simulink model "simulink_test1"  (R2014a)
settings: Solver=ode45  StartTime=0.0  StopTime=10.0  RelTol=1e-3
values from neighbouring files (symbols this model uses):
  Gb = 200    [pole_placement.m]    (also in pole_placement2.m; time_domain.m)
  Ib = 0    [pole_placement.m]    (also in pole_placement2.m; time_domain.m)
  n = 0.142    [pole_placement.m]    (also in pole_placement2.m; time_domain.m)
  p1 = 0.035    [pole_placement.m]    (also in pole_placement2.m; time_domain.m)
  p2 = 0.05    [pole_placement.m]    (also in pole_placement2.m; time_domain.m)
  p3 = 0.000023    (= 2.3e-05)    [pole_placement.m]    (also in pole_placement2.m = 2.8e-05; time_domain.m)
  VG = 117    [pole_placement.m]    (also in pole_placement2.m; time_domain.m)
  VI = 1/0.098    (= 10.2040816327)    [pole_placement.m]    (also in pole_placement2.m; time_domain.m)
undefined symbols (not defined in the file or in its folder): Ge, k1, k2, k3, kr, l1, l2, l3, r, Vg, Xe
settings Model: Creator=joach  LastModifiedBy=joach
settings OptimizationCC: SimCompilerOptimization=off
settings DebuggingCC: MergeDetectMultiDrivingBlocksExec=error  FrameProcessingCompatibilityMsg=error
settings RTWCC: RTWCompilerOptimization=off
settings ConfigComp: CovMetricSettings=dw  CovHtmlReporting=on  CovSaveCumulativeToWorkspaceVar=on  CovSaveSingleToWorkspaceVar=on  CovModelRefEnable=Off  CovExternalEMLEnable=off  CovSFcnEnable=off

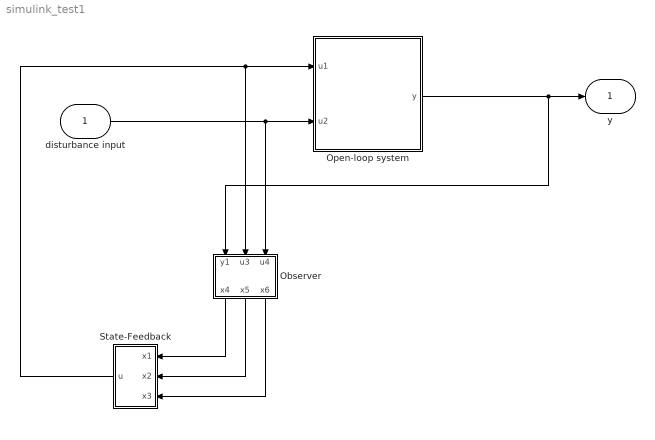
== system simulink_test1 ==
  disturbance input : Inport
  Observer : Subsystem
  Open-loop system : Subsystem
  State-Feedback : Subsystem
  y : Outport
  wires:
  disturbance input/1 -> Open-loop system/2(u2), Observer/3(u4)
  Observer/2(x5) -> State-Feedback/2(x2)
  Observer/3(x6) -> State-Feedback/3(x3)
  Open-loop system/1(y) -> Observer/1(y1), y/1
  State-Feedback/1(u) -> Open-loop system/1(u1), Observer/2(u3)
  Observer/1(x4) -> State-Feedback/1(x1)

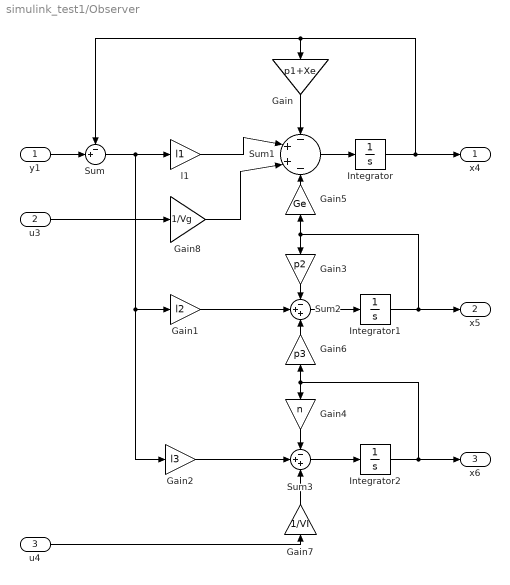
== system simulink_test1/Observer ==
  y1 : Inport
  u3 : Inport  Port=2
  u4 : Inport  Port=3
  Gain : Gain  Gain=p1+Xe
  Gain1 : Gain  Gain=l2
  Gain2 : Gain  Gain=l3
  Gain3 : Gain  Gain=p2
  Gain4 : Gain  Gain=n
  Gain5 : Gain  Gain=Ge
  Gain6 : Gain  Gain=p3
  Gain7 : Gain  Gain=1/VI
  Gain8 : Gain  Gain=1/Vg
  Integrator : Integrator
  Integrator1 : Integrator
  Integrator2 : Integrator
  Sum : Sum  Inputs=-+|
  Sum1 : Sum  Inputs=-++-
  Sum2 : Sum  Inputs=-++
  Sum3 : Sum  Inputs=-++
  l1 : Gain  Gain=l1
  x4 : Outport
  x5 : Outport  Port=2
  x6 : Outport  Port=3
  wires:
  Sum/1 -> Gain2/1, Gain1/1, l1/1
  Sum1/1 -> Integrator/1
  l1/1 -> Sum1/2
  Integrator/1 -> x4/1, Sum/1, Gain/1
  Gain2/1 -> Sum3/2
  Gain1/1 -> Sum2/2
  Integrator1/1 -> x5/1, Gain5/1, Gain3/1
  y1/1 -> Sum/2
  Gain/1 -> Sum1/1
  Sum2/1 -> Integrator1/1
  Integrator2/1 -> x6/1, Gain6/1, Gain4/1
  Gain3/1 -> Sum2/1
  Sum3/1 -> Integrator2/1
  Gain7/1 -> Sum3/3
  Gain4/1 -> Sum3/1
  Gain6/1 -> Sum2/3
  u3/1 -> Gain8/1
  Gain5/1 -> Sum1/4
  Gain8/1 -> Sum1/3
  u4/1 -> Gain7/1

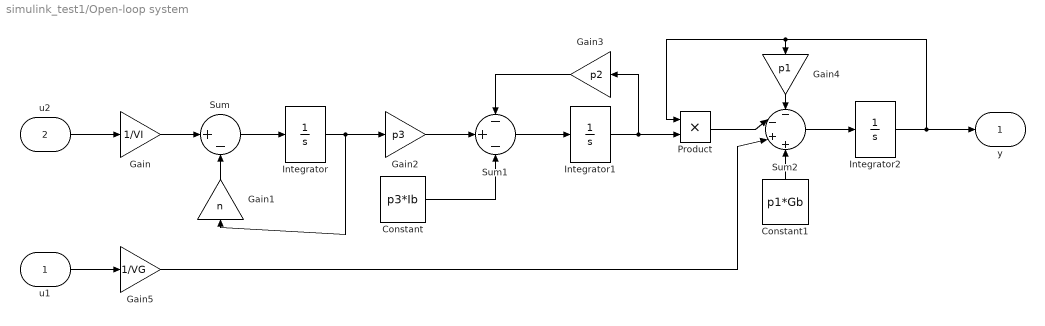
== system simulink_test1/Open-loop system ==
  u1 : Inport
  u2 : Inport  Port=2
  " Gain" : Gain  Gain=1/VI
  " Gain2" : Gain  Gain=p3
  " Gain3" : Gain  Gain=p2
  " Gain4" : Gain  Gain=p1
  " Gain5" : Gain  Gain=1/VG
  Constant : Constant  Value=p3*Ib
  Constant1 : Constant  Value=p1*Gb
  Gain1 : Gain  Gain=n
  Integrator : Integrator
  Integrator1 : Integrator
  Integrator2 : Integrator
  Product : Product
  Sum : Sum  Inputs=|+-
  Sum1 : Sum  Inputs=-+-
  Sum2 : Sum  Inputs=--++
  y : Outport
  wires:
  " Gain4"/1 -> Sum2/1
  Integrator1/1 -> " Gain3"/1, Product/2
  " Gain5"/1 -> Sum2/3
  Constant/1 -> Sum1/3
  Sum/1 -> Integrator/1
  " Gain2"/1 -> Sum1/2
  Sum1/1 -> Integrator1/1
  Gain1/1 -> Sum/2
  " Gain3"/1 -> Sum1/1
  Product/1 -> Sum2/2
  Integrator/1 -> Gain1/1, " Gain2"/1
  Integrator2/1 -> y/1, " Gain4"/1, Product/1
  Sum2/1 -> Integrator2/1
  " Gain"/1 -> Sum/1
  Constant1/1 -> Sum2/4
  u1/1 -> " Gain5"/1
  u2/1 -> " Gain"/1

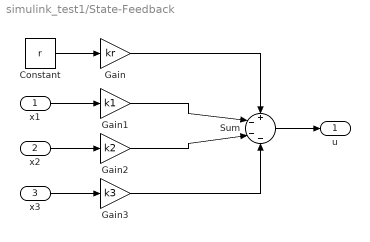
== system simulink_test1/State-Feedback ==
  x1 : Inport
  x2 : Inport  Port=2
  x3 : Inport  Port=3
  Constant : Constant  Value=r
  Gain : Gain  Gain=kr
  Gain1 : Gain  Gain=k1
  Gain2 : Gain  Gain=k2
  Gain3 : Gain  Gain=k3
  Sum : Sum  Inputs=+---
  u : Outport
  wires:
  Gain1/1 -> Sum/2
  x2/1 -> Gain2/1
  x3/1 -> Gain3/1
  Constant/1 -> Gain/1
  Gain/1 -> Sum/1
  Gain2/1 -> Sum/3
  Sum/1 -> u/1
  Gain3/1 -> Sum/4
  x1/1 -> Gain1/1
